simulink model "BodyModel_Simulink"  (R2021a)
settings: Solver=ode23tb  StartTime=0.0  StopTime=12.36  RelTol=1e-3
undefined symbols (not defined in the file): A_m, B_m, C_m, D_m, K_lqr, QuadrotorBodyModel_Object, u_ss, x_des
libraries: dspsigattribs x1, uavutilslib x1
settings Model: OrderedModelArguments=off  Creator=prenk  LastModifiedBy=renkert2
settings SolverCC: AlgebraicLoopSolver=TrustRegion
settings DebuggingCC: SFMachineParentedDataDiag=warning

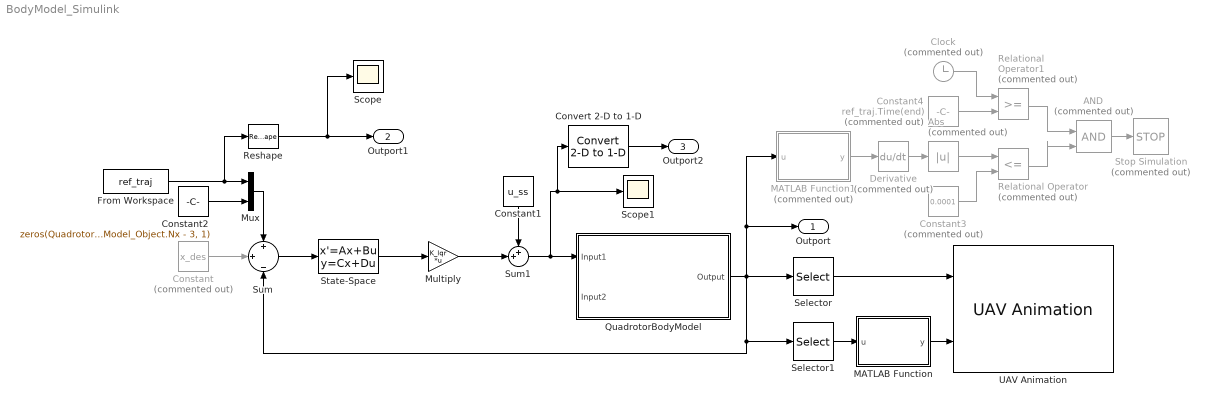
== system BodyModel_Simulink ==
  AND : Logic  Commented=on  IconShape=distinctive  AllPortsSameDT=off  OutDataTypeStr=boolean
  Abs : Abs  Commented=on
  Clock : Clock  Commented=on
  Constant : Constant  Commented=on  Value=x_des  VectorParams1D=off
  Constant1 : Constant  Value=u_ss
  Constant2 : Constant  Value=zeros(QuadrotorBodyModel_Object.Nx - 3, 1)
  Constant3 : Constant  Commented=on  Value=0.0001
  Constant4 : Constant  Commented=on  Value=ref_traj.Time(end)
  Convert 2-D to 1-D : dspsigattribs/Convert 2-D to 1-D
      settings: SourceProductBaseCode=DS
  Derivative : Derivative  Commented=on  CoefficientInTFapproximation=100
  From Workspace : FromWorkspace  VariableName=ref_traj  OutputAfterFinalValue=Holding final value
  MATLAB Function : MATLAB Function  TreatAsAtomicUnit=on
  MATLAB Function1 : MATLAB Function  Commented=on  TreatAsAtomicUnit=on
  Multiply : Gain  Gain=K_lqr  Multiplication=Matrix(K*u)
  Mux : Mux  Inputs=2
  QuadrotorBodyModel : Subsystem  mask{x_0=QuadrotorBodyModel_Object.x0}
  Relational Operator : RelationalOperator  Commented=on  Operator=<=  OutDataTypeStr=boolean  RndMeth=Simplest
  Relational Operator1 : RelationalOperator  Commented=on  OutDataTypeStr=boolean  RndMeth=Simplest
  Reshape : Reshape
  Scope : Scope
  Scope1 : Scope
  Selector : Selector  InputPortWidth=QuadrotorBodyModel_Object.Nx  IndexOptions=Index vector (dialog)  Indices=QuadrotorBodyModel_Object.I.x.p  OutputSizes=1
  Selector1 : Selector  InputPortWidth=QuadrotorBodyModel_Object.Nx  IndexOptions=Index vector (dialog)  Indices=QuadrotorBodyModel_Object.I.x.Theta  OutputSizes=1
  State-Space : StateSpace  A=A_m  B=B_m  C=C_m  D=D_m  InitialCondition=0
  Stop Simulation : Stop  Commented=on
  Sum : Sum  Inputs=+|+|-
  Sum1 : Sum  Inputs=++|
  UAV Animation : uavutilslib/UAV Animation  UAVType=Multirotor  UAVSize=1  InertialZDirection=Down  SampleTime=-1
      settings: SourceProductBaseCode=UV
  Outport : Outport  SignalName=y_out
  Outport1 : Outport  Port=2  SignalName=r_out
  Outport2 : Outport  Port=3  SignalName=u_out
  wires:
  Constant/1 -> Sum/2
  Constant1/1 -> Sum1/1
  Sum1/1 -> Convert 2-D to 1-D/1, Scope1/1, QuadrotorBodyModel/1(Input1)
  Multiply/1 -> Sum1/2
  Sum/1 -> State-Space/1
  State-Space/1 -> Multiply/1
  Mux/1 -> Sum/1
  Constant2/1 -> Mux/2
  Abs/1 -> Relational Operator/1
  Constant3/1 -> Relational Operator/2
  MATLAB Function1/1(y) -> Derivative/1
  Relational Operator/1 -> AND/2
  Clock/1 -> Relational Operator1/1
  Constant4/1 -> Relational Operator1/2
  Relational Operator1/1 -> AND/1
  AND/1 -> Stop Simulation/1
  Derivative/1 -> Abs/1
  From Workspace/1 -> Reshape/1, Mux/1
  Reshape/1 -> Scope/1, Outport1/1
  MATLAB Function/1(y) -> UAV Animation/2
  Selector1/1 -> MATLAB Function/1(u)
  Selector/1 -> UAV Animation/1
  QuadrotorBodyModel/1(Output) -> Selector1/1, Sum/3, Outport/1, MATLAB Function1/1(u), Selector/1
  Convert 2-D to 1-D/1 -> Outport2/1

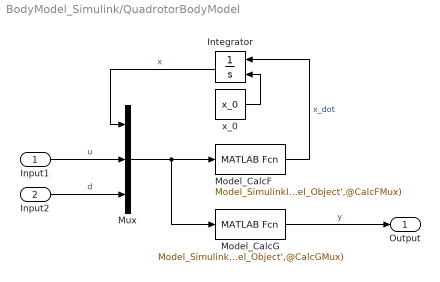
== system BodyModel_Simulink/QuadrotorBodyModel ==
  Input1 : Inport  PortDimensions=[QuadrotorBodyModel_Object.Nu,1]
  Input2 : Inport  Port=2  PortDimensions=[QuadrotorBodyModel_Object.Nd,1]
  Integrator : Integrator  InitialConditionSource=external
  Model_CalcF : MATLABFcn  MATLABFcn=Model_SimulinkInterpretedFunction(u,'BodyModel_Simulink','QuadrotorBodyModel_Object',@CalcFMux)  OutputDimensions=QuadrotorBodyModel_Object.Nx
  Model_CalcG : MATLABFcn  MATLABFcn=Model_SimulinkInterpretedFunction(u,'BodyModel_Simulink','QuadrotorBodyModel_Object',@CalcGMux)  OutputDimensions=QuadrotorBodyModel_Object.Ny
  Mux : Mux  Inputs=3
  x_0 : Constant  Value=x_0  VectorParams1D=off
  Output : Outport
  wires:
  Model_CalcF/1 -> Integrator/1  "x_dot"
  Input1/1 -> Mux/2  "u"
  Model_CalcG/1 -> Output/1  "y"
  x_0/1 -> Integrator/2
  Input2/1 -> Mux/3  "d"
  Integrator/1 -> Mux/1  "x"
  Mux/1 -> Model_CalcG/1, Model_CalcF/1

== matlab function BodyModel_Simulink/MATLAB Function ==
  data: u input; y output
function y = eul2quatMF(u)
    y = eul2quat([1 -1 1].*fliplr(u'),'ZYX');
end

== matlab function BodyModel_Simulink/MATLAB Function1 ==
  data: u input; y output
function y = vecnorm(u)

y = norm(u,2);
end
